simulink model "Model"  (R2018b)
settings: Solver=ode45  StartTime=0.0  StopTime=30  RelTol=1e-3  EnableMultiTasking=on
values from neighbouring files (symbols this model uses):
  A = [0 1 0 0 0 0 0; a21 a22 a23 a24 a25 0 0; 0 a32 a33 0 0 0 0;0 0 0 0 1 0 0;a51 a52 0 a54 a55 a56 0; 0 0 0 0 0 0 1;0 0 0 a74 0 a76 0]    [Main.m]
  B = [ 0; 0; b31; 0; 0; 0; 0]    [Main.m]
  C = [1 1 1 1 1 1 1]'    [Main.m]
  E = [0; 0; 0; 0; e51; 0; e71]    [Main.m]
  Kkr = 3729    [Main.m]
  Tkr = 26.736e-3    (= 0.026736)    [Main.m]
  Umax = 24    [Main.m]
settings Model: Creator=Ervin  LastModifiedBy=Ervin
settings DataIOCC: LimitDataPoints=on  SaveFormat=Array
settings OptimizationCC: LifeSpan=inf
settings DebuggingCC: IgnoredZcDiagnostic=none  SFUnexpectedBacktrackingDiag=warning  SFNoUnconditionalDefaultTransitionDiag=warning  SFExecutionAtInitializationDiag=none
settings HardwareCC: ProdBitPerPointer=32  ProdBitPerSizeT=32  ProdBitPerPtrDiffT=32  ProdLargestAtomicFloat=None  ProdIntDivRoundTo=Undefined  ProdEndianess=Unspecified  ProdWordSize=32  ProdHWDeviceType=32-bit Generic
settings ModelReferenceCC: PropagateSignalLabelsOutOfModel=off
settings SFSimCC: SimUseLocalCustomCode=off
settings RTWCC: RTWUseLocalCustomCode=off
settings CodeAppCC: StateflowObjectComments=on
settings GRTTargetCC: TargetLangStandard=C89/C90 (ANSI)  GeneratePreprocessorConditionals=Disable all
settings ConfigComp: CovMetricSettings=dw  CovHtmlReporting=on  CovSaveCumulativeToWorkspaceVar=on  CovSaveSingleToWorkspaceVar=on  CovExternalEMLEnable=off

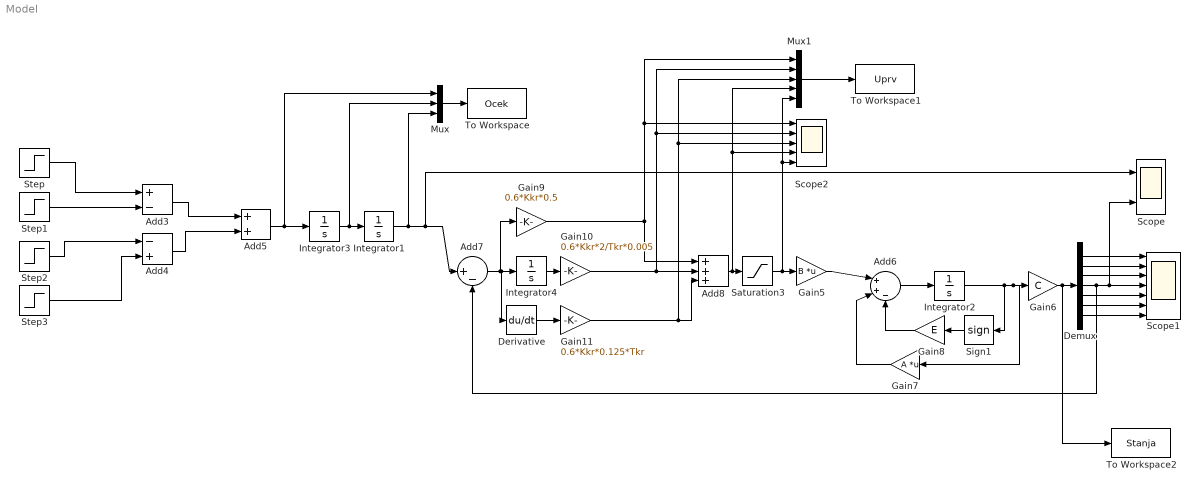
== system Model ==
  Add3 : Sum  Inputs=+-
  Add4 : Sum  Inputs=-+
  Add5 : Sum
  Add6 : Sum  Inputs=|++-
  Add7 : Sum  Inputs=|+-
  Add8 : Sum  Inputs=+++
  Demux : Demux  Outputs=7
  Derivative : Derivative  CoefficientInTFapproximation=1/100
  Gain10 : Gain  Gain=0.6*Kkr*2/Tkr*0.005
  Gain11 : Gain  Gain=0.6*Kkr*0.125*Tkr
  Gain5 : Gain  Gain=B  Multiplication=Matrix(K*u)
  Gain6 : Gain  Gain=C
  Gain7 : Gain  Gain=A  Multiplication=Matrix(K*u)
  Gain8 : Gain  Gain=E
  Gain9 : Gain  Gain=0.6*Kkr*0.5
  Integrator{1..4} (4 alike) : Integrator
  Mux : Mux  Inputs=3
  Mux1 : Mux  Inputs=5
  Saturation3 : Saturate  UpperLimit=Umax  LowerLimit=-Umax  ZeroCross=off
  Scope : Scope  NumInputPorts=2
  Scope1 : Scope  NumInputPorts=7
  Scope2 : Scope  NumInputPorts=5
  Sign1 : Signum  ZeroCross=off
  Step : Step  Time=0  After=20/27  SampleTime=0
  Step1 : Step  Time=0.15  After=20/27  SampleTime=0
  Step2 : Step  Time=1.35  After=20/27  SampleTime=0
  Step3 : Step  Time=1.5  After=20/27  SampleTime=0
  To Workspace : ToWorkspace  VariableName=Ocek  SaveFormat=Structure With Time  SampleTime=-1
  To Workspace1 : ToWorkspace  VariableName=Uprv  SaveFormat=Structure With Time  SampleTime=-1
  To Workspace2 : ToWorkspace  VariableName=Stanja  SaveFormat=Structure With Time  SampleTime=-1
  wires:
  Step3/1 -> Add4/2
  Step/1 -> Add3/1
  Add4/1 -> Add5/2
  Step2/1 -> Add4/1
  Add5/1 -> Mux/1, Integrator3/1
  Add3/1 -> Add5/1
  Step1/1 -> Add3/2
  Integrator3/1 -> Mux/2, Integrator1/1
  Sign1/1 -> Gain8/1
  Gain7/1 -> Add6/2
  Gain8/1 -> Add6/3
  Integrator1/1 -> Mux/3, Scope/1, Add7/1
  Saturation3/1 -> Scope2/5, Mux1/5, Gain5/1
  Gain5/1 -> Add6/1
  Integrator2/1 -> Sign1/1, Gain7/1, Gain6/1
  Add6/1 -> Integrator2/1
  Integrator4/1 -> Gain10/1
  Add7/1 -> Derivative/1, Integrator4/1, Gain9/1
  Add8/1 -> Scope2/4, Mux1/4, Saturation3/1
  Gain11/1 -> Scope2/3, Mux1/3, Add8/3
  Derivative/1 -> Gain11/1
  Demux/4 -> Scope1/4, Scope/2, Add7/2
  Gain9/1 -> Add8/1, Scope2/1, Mux1/1
  Gain10/1 -> Scope2/2, Mux1/2, Add8/2
  Gain6/1 -> To Workspace2/1, Demux/1
  Demux/1 -> Scope1/1
  Demux/2 -> Scope1/2
  Demux/3 -> Scope1/3
  Demux/5 -> Scope1/5
  Demux/6 -> Scope1/6
  Demux/7 -> Scope1/7
  Mux/1 -> To Workspace/1
  Mux1/1 -> To Workspace1/1
